simulink model "a5nl_sw_subsystem_lsg"  (R2020b)
settings: Solver=ode45  StartTime=0.0  StopTime=10.0  MaxStep=0.01  RelTol=1e-3  EnableMultiTasking=on
values from neighbouring files (symbols this model uses):
  c = 0.1    [a3Scr_lsg.m]
  k = 1    [a3Scr_lsg.m]
  m = 2    [a3Scr_lsg.m]
  v0 = 0    [a3Scr_lsg.m]
  y0 = 3    [a3Scr_lsg.m]
settings Model: Creator=Reichl  LastModifiedBy=jakob
settings DataIOCC: LimitDataPoints=on  SaveFormat=Array  SignalLoggingSaveFormat=ModelDataLogs  ReturnWorkspaceOutputs=off
settings OptimizationCC: ExpressionDepthLimit=2147483647  LifeSpan=inf
settings DebuggingCC: UnderspecifiedInitializationDetection=Classic  MergeDetectMultiDrivingBlocksExec=none  SolverPrmCheckMsg=warning  FcnCallInpInsideContextMsg=warning  StateNameClashWarn=warning  SFUnexpectedBacktrackingDiag=warning  SFNoUnconditionalDefaultTransitionDiag=warning  SFExecutionAtInitializationDiag=none  ArithmeticOperatorsInVariantConditions=warning
settings HardwareCC: ProdBitPerPointer=32  ProdBitPerSizeT=32  ProdBitPerPtrDiffT=32  ProdLargestAtomicFloat=None  ProdIntDivRoundTo=Undefined  ProdEndianess=Unspecified  ProdWordSize=32  ProdHWDeviceType=32-bit Generic
settings ModelReferenceCC: PropagateSignalLabelsOutOfModel=off
settings SFSimCC: SimUseLocalCustomCode=off  CustomCodeUndefinedFunction=UseInterfaceOnly
settings RTWCC: RTWUseLocalCustomCode=off
settings CodeAppCC: StateflowObjectComments=on
settings GRTTargetCC: TargetLangStandard=C89/C90 (ANSI)  CombineOutputUpdateFcns=off  GRTInterface=on
settings ConfigComp: CovMetricSettings=dw  CovSaveCumulativeToWorkspaceVar=on  CovSaveSingleToWorkspaceVar=on  CovExternalEMLEnable=off  CovSFcnEnable=off

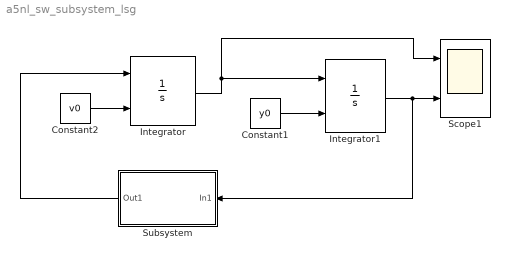
== system a5nl_sw_subsystem_lsg ==
  Constant1 : Constant  Value=y0
  Constant2 : Constant  Value=v0
  Integrator : Integrator  InitialConditionSource=external
  Integrator1 : Integrator  InitialConditionSource=external  InitialCondition=3
  Scope1 : Scope  NumInputPorts=2
  Subsystem : Subsystem
  wires:
  Integrator/1 -> Integrator1/1, Scope1/1
  Subsystem/1(Out1) -> Integrator/1
  Constant2/1 -> Integrator/2
  Constant1/1 -> Integrator1/2
  Integrator1/1 -> Scope1/2, Subsystem/1(In1)

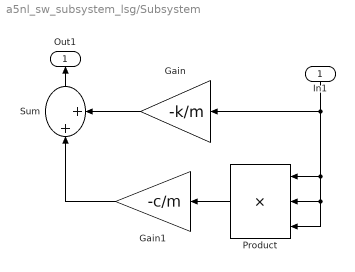
== system a5nl_sw_subsystem_lsg/Subsystem ==
  In1 : Inport
  Gain : Gain  Gain=-k/m
  Gain1 : Gain  Gain=-c/m
  Product : Product  Inputs=***  RndMeth=Zero
  Sum : Sum  Inputs=|++
  Out1 : Outport  VectorParamsAs1DForOutWhenUnconnected=off
  wires:
  Gain/1 -> Sum/2
  Product/1 -> Gain1/1
  Gain1/1 -> Sum/1
  In1/1 -> Product/3, Product/2, Product/1, Gain/1
  Sum/1 -> Out1/1
